simulink model "bldc_2016_mamf"  (R2022b)
settings: Solver=FixedStepAuto  StartTime=0.0  StopTime=t_max  FixedStep=timestep  RelTol=1e-3
values from neighbouring files (symbols this model uses):
  den = [1 ((L*D+R*J)/(L*J)) Kt*Kb/(L*J)]    [script.m]
  num = Kt*Kb/(L*J)    (= 39490.1730769)    [script.m]
  step_v = 1000    [script.m]
settings Model: Creator=ricar  LastModifiedBy=mluser
settings SolverCC: AlgebraicLoopSolver=TrustRegion
settings DataIOCC: ReturnWorkspaceOutputs=off
settings DebuggingCC: UnconnectedInputMsg=warning  UnconnectedOutputMsg=warning  UnconnectedLineMsg=warning  SFMachineParentedDataDiag=warning  ArithmeticOperatorsInVariantConditions=warning
settings ModelReferenceCC: EnableRefExpFcnMdlSchedulingChecks=on
settings SFSimCC: SimUseLocalCustomCode=off  CustomCodeUndefinedFunction=UseInterfaceOnly
settings RTWCC: RTWUseLocalCustomCode=off
settings CodeAppCC: StateflowObjectComments=on

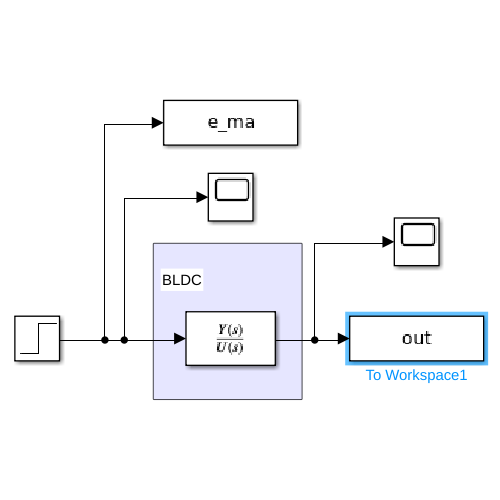
[thumbnail: Simulink's stored preview of the top-level diagram]
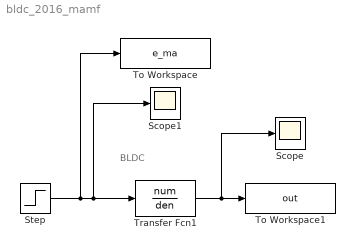
== system bldc_2016_mamf ==
  note: BLDC
  Scope : Scope
  Scope1 : Scope
  Step : Step  Time=0  After=step_v  SampleTime=0
  To Workspace : ToWorkspace  VariableName=e_ma  SampleTime=-1
  To Workspace1 : ToWorkspace  VariableName=out  SampleTime=-1
  Transfer Fcn1 : TransferFcn  Numerator=num  Denominator=den
  wires:
  Step/1 -> Transfer Fcn1/1, Scope1/1, To Workspace/1
  Transfer Fcn1/1 -> To Workspace1/1, Scope/1
